simulink model "Backstep"  (R2015a)
settings: Solver=ode45  StartTime=0.0  StopTime=10.0  RelTol=1e-3
values from neighbouring files (symbols this model uses):
  a1 = (Iy-Iz)/Ix    (= -0.371382636656)    [Donnees_quadri.m]
  a2 = Irotor/Ix    (= 9.6463022508e-05)    [Donnees_quadri.m]
  a3 = (Iz-Ix)/Iy    (= 0.466575716235)    [Donnees_quadri.m]
  a4 = Irotor/Iy    (= 8.18553888131e-05)    [Donnees_quadri.m]
  a5 = (Ix-Iy)/Iz    (= -0.115145228216)    [Donnees_quadri.m]
  b1 = L/Ix    (= 16.077170418)    [Donnees_quadri.m]
  b2 = L/Iy    (= 13.6425648022)    [Donnees_quadri.m]
  b3 = L/Iz    (= 10.3734439834)    [Donnees_quadri.m]
  c1 = 5.52    [Donnees_quadri.m]
  c2 = 3.4    [Donnees_quadri.m]
  c3 = 1    [Donnees_quadri.m]
  c4 = 1    [Donnees_quadri.m]
  c5 = 3.07    [Donnees_quadri.m]
  c6 = 4.71    [Donnees_quadri.m]
  c7 = 6.11    [Donnees_quadri.m]
  c8 = 7.96    [Donnees_quadri.m]
  g = 9.81    [Donnees_quadri.m]
  m = 0.65    [Donnees_quadri.m]
  phi_dot_d = 0    [Donnees_quadri.m]
  psi_d = 2    [Donnees_quadri.m]
  psi_dot_d = 0    [Donnees_quadri.m]
  theta_dot_d = 0    [Donnees_quadri.m]
  x_dot_dot_d = 0    [Donnees_quadri.m]
  y_dot_dot_d = 0    [Donnees_quadri.m]
  z_d = 5    [Donnees_quadri.m]
  z_dot_d = 0    [Donnees_quadri.m]
settings Model: Creator=Lenovo  LastModifiedBy=Lenovo

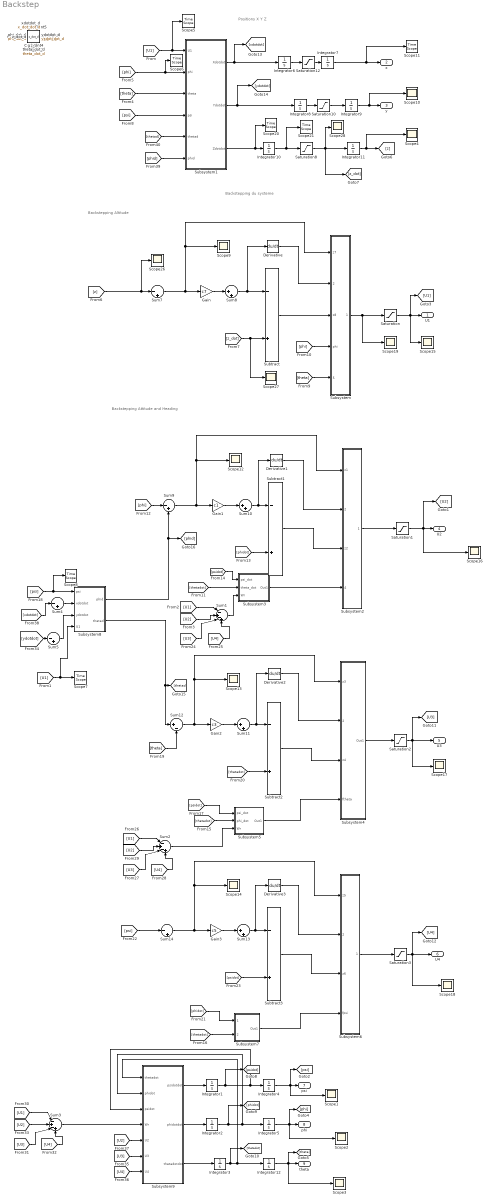
== system Backstep ==
  note: Positions X Y Z
  note: Backstepping Altitude
  note: Backstepping du systeme
  note: Backstepping Attitude and Heading
  Derivative{,1..3} (4 alike) : Derivative
  Gain : Gain  Gain=c7
  Gain1 : Gain  Gain=c1
  Gain2 : Gain  Gain=c3
  Gain3 : Gain  Gain=c5
  Integrator{1..12} (12 alike) : Integrator
  Saturation : Saturate  UpperLimit=500  LowerLimit=-500
  Saturation{1..3,8,10,12} (6 alike) : Saturate  UpperLimit=5  LowerLimit=-5
  Scope{1..4,9..10,12..19,26..28} (17 alike) : Scope
      Scope10 settings: SaveName=ScopeData9
      Scope12 settings: SaveName=ScopeData11
      Scope13 settings: SaveName=ScopeData12
      Scope14 settings: SaveName=ScopeData13
      Scope15 settings: SaveName=ScopeData14
      Scope16 settings: SaveName=ScopeData15
      Scope17 settings: SaveName=ScopeData16
      Scope18 settings: SaveName=ScopeData17
      Scope19 settings: SaveName=ScopeData24
      Scope2 settings: SaveName=ScopeData3
      Scope26 settings: SaveName=ScopeData39
      Scope27 settings: SaveName=ScopeData45
      Scope28 settings: SaveName=ScopeData46
      Scope3 settings: SaveName=ScopeData4
      Scope4 settings: SaveName=ScopeData2
      Scope9 settings: SaveName=ScopeData8
  Scope{5..8,11,20..21} (7 alike) : TimeScope
  Subsystem : Subsystem
  Subsystem1 : Subsystem
  Subsystem2 : Subsystem
  Subsystem3 : Subsystem
  Subsystem4 : Subsystem
  Subsystem5 : Subsystem
  Subsystem6 : Subsystem
  Subsystem7 : Subsystem
  Subsystem8 : Subsystem
  Subsystem9 : Subsystem
  Subtract{,1..3} (4 alike) : Sum  Inputs=-+
  Sum1 : Sum  Inputs=|-+-+
  Sum{8,10..11,13} (4 alike) : Sum  Inputs=|++
  Sum12 : Sum  Inputs=|+-
  Sum{4..5,7,9,14} (5 alike) : Sum  Inputs=|-+
  Sum2 : Sum  Inputs=|-+-+
  Sum3 : Sum  Inputs=|-+-+
  U1 : Outport
  x : Outport  Port=2
  y : Outport  Port=3
  U2 : Outport  Port=4
  U3 : Outport  Port=5
  U4 : Outport  Port=6
  psi : Outport  Port=7
  phi : Outport  Port=8
  "theta " : Outport  Port=9
  1 : Constant  IOType=siggen
  Constant : Constant  IOType=siggen
  Constant1 : Constant  IOType=siggen  Value=a4
  Constant2 : Constant  IOType=siggen  Value=a3
  Constant3 : Constant  IOType=siggen  Value=a2
  Constant4 : Constant  IOType=siggen  Value=a1
  Constant5 : Constant  IOType=siggen  Value=a5
  a1 : Constant  IOType=siggen  Value=a1
  a2 : Constant  IOType=siggen  Value=a2
  a3 : Constant  IOType=siggen  Value=a3
  a4 : Constant  IOType=siggen  Value=a4
  a5 : Constant  IOType=siggen  Value=a5
  b1 : Constant  IOType=siggen  Value=b1
  b2 : Constant  IOType=siggen  Value=b2
  b3 : Constant  IOType=siggen  Value=b3
  c2 : Constant  IOType=siggen  Value=c2
  c4 : Constant  IOType=siggen  Value=c4
  c6 : Constant  IOType=siggen  Value=c6
  c8 : Constant  IOType=siggen  Value=c8
  g : Constant  IOType=siggen  Value=g
  m : Constant  IOType=siggen  Value=m
  phi_dot_d : Constant  IOType=siggen  Value=phi_dot_d
  psi_d : Constant  IOType=siggen  Value=psi_d
  psi_dot_d : Constant  IOType=siggen  Value=psi_dot_d
  theta_dot_d : Constant  IOType=siggen  Value=theta_dot_d
  xdotdot_d : Constant  IOType=siggen  Value=x_dot_dot_d
  ydotdot_d : Constant  IOType=siggen  Value=y_dot_dot_d
  z_d : Constant  IOType=siggen  Value=z_d
  z_dot_d : Constant  IOType=siggen  Value=z_dot_d
  wires:
  Sum7/1 -> Scope9/1, Subsystem/1(z7), Gain/1
  Subtract/1 -> Subsystem/3(z8)
  Subsystem/1(Out1) -> Scope19/1, Saturation/1
  Gain/1 -> Sum8/1
  Sum8/1 -> Derivative/1, Subtract/1
  Saturation/1 -> [U1], Scope15/1, U1/1
  [U1] -> Scope5/1, Subsystem1/1(U1)
  Integrator6/1 -> Saturation12/1
  Integrator8/1 -> Saturation10/1
  Integrator10/1 -> Scope21/1, Saturation8/1
  Integrator11/1 -> Scope4/1, [z]
  [z] -> Scope26/1, Sum7/1
  Integrator9/1 -> Scope10/1, y/1
  Integrator7/1 -> Scope11/1, x/1
  Sum9/1 -> Scope12/1, Subsystem2/1(z1), Gain1/1
  Subtract1/1 -> Subsystem2/3(z2)
  Subsystem2/1(Out1) -> Saturation1/1
  Gain1/1 -> Sum10/1
  Sum10/1 -> Derivative1/1, Subtract1/1
  Saturation1/1 -> [U2], Scope16/1, U2/1
  Subsystem3/1(Out1) -> Subsystem2/4(fphi)
  [z_dot] -> Scope27/1, Subtract/2
  Sum12/1 -> Scope13/1, Subsystem4/1(z3), Gain2/1
  Subtract2/1 -> Subsystem4/3(z4)
  Subsystem4/1(Out1) -> Saturation2/1
  Gain2/1 -> Sum11/1
  Sum11/1 -> Derivative2/1, Subtract2/1
  Saturation2/1 -> [U3], Scope17/1, U3/1
  [psidot] -> Subsystem5/1(psi_dot)
  Subsystem5/1(Out1) -> Subsystem4/4(ftheta)
  [thetadot] -> Subtract2/2
  Sum14/1 -> Scope14/1, Subsystem6/1(z5), Gain3/1
  Subtract3/1 -> Subsystem6/3(z6)
  Subsystem6/1(Out1) -> Saturation3/1
  Gain3/1 -> Sum13/1
  Sum13/1 -> Derivative3/1, Subtract3/1
  Saturation3/1 -> [U4], U4/1, Scope18/1
  [phidot] -> Subsystem7/1(phi_dot)
  [thetadot] -> Subsystem7/2(theta_dot)
  Subsystem7/1(Out1) -> Subsystem6/4(fpsi)
  [psidot] -> Subtract3/2
  [phidot] -> Subtract1/2
  [theta] -> Subsystem/5(theta)
  Derivative/1 -> Subsystem/2(zdd_d+c7zd_d-c7zd)
  [phi] -> Subsystem/4(phi)
  Derivative1/1 -> Subsystem2/2(phidd_d+c1phid_d-c1phid)
  Derivative2/1 -> Subsystem4/2(thetadd_d+c3thetad_d-c3thetad)
  Derivative3/1 -> Subsystem6/2(psidd_d+c5psid_d-c5psid)
  Subsystem1/3(Zdotdot) -> Scope20/1, Integrator10/1
  Saturation8/1 -> Scope28/1, [z_dot], Integrator11/1
  Saturation10/1 -> Integrator9/1
  Subsystem1/2(Ydotdot) -> Integrator8/1, [ydotdot]
  Subsystem1/1(Xdotdot) -> Integrator6/1, [xdotdot]
  Saturation12/1 -> Integrator7/1
  [psi] -> Scope8/1, Subsystem8/1(psi)
  Subsystem8/1(phid) -> [phid], Sum9/2
  Subsystem8/2(thetad) -> [thetad], Sum12/1
  [U1] -> Subsystem8/4(U1), Scope7/1
  [thetadot] -> Subsystem5/2(phi_dot)
  [phi] -> Sum9/1
  [theta] -> Subsystem1/3(theta)
  [psi] -> Subsystem1/4(psi)
  [phi] -> Scope6/1, Subsystem1/2(phi)
  [U1] -> Sum1/1
  Sum1/1 -> Subsystem3/3(Wr)
  [U2] -> Sum1/2
  Subsystem9/2(phidotdot) -> Integrator2/1
  Subsystem9/1(psidotdot) -> Integrator1/1
  Subsystem9/3(thetadotdot) -> Integrator3/1
  Integrator4/1 -> Scope1/1, [psi], psi/1
  Integrator5/1 -> Scope2/1, [phi], phi/1
  Integrator12/1 -> Scope3/1, [theta], "theta "/1
  Integrator1/1 -> [psidot], Subsystem9/3(psidot), Integrator4/1
  Integrator2/1 -> [phidot], Subsystem9/2(phidot), Integrator5/1
  Integrator3/1 -> [thetadot], Subsystem9/1(thetadot), Integrator12/1
  [psidot] -> Subsystem3/1(psi_dot)
  [thetadot] -> Subsystem3/2(theta_dot)
  [theta] -> Sum12/2
  [psi] -> Sum14/1
  [U3] -> Sum1/3
  [U4] -> Sum1/4
  [U1] -> Sum2/1
  Sum2/1 -> Subsystem5/3(Wr)
  [U2] -> Sum2/2
  [U3] -> Sum2/3
  [U4] -> Sum2/4
  [U1] -> Sum3/1
  [U2] -> Sum3/2
  [U3] -> Sum3/3
  [U4] -> Sum3/4
  Sum3/1 -> Subsystem9/4(Wr)
  [U2] -> Subsystem9/5(U2)
  [U3] -> Subsystem9/6(U3)
  [U4] -> Subsystem9/7(U4)
  [thetad] -> Subsystem1/5(thetad)
  [phid] -> Subsystem1/6(phid)
  Sum4/1 -> Subsystem8/2(xdotdot)
  [ydotdot] -> Sum5/1
  Sum5/1 -> Subsystem8/3(ydotdot)
  [xdotdot] -> Sum4/1

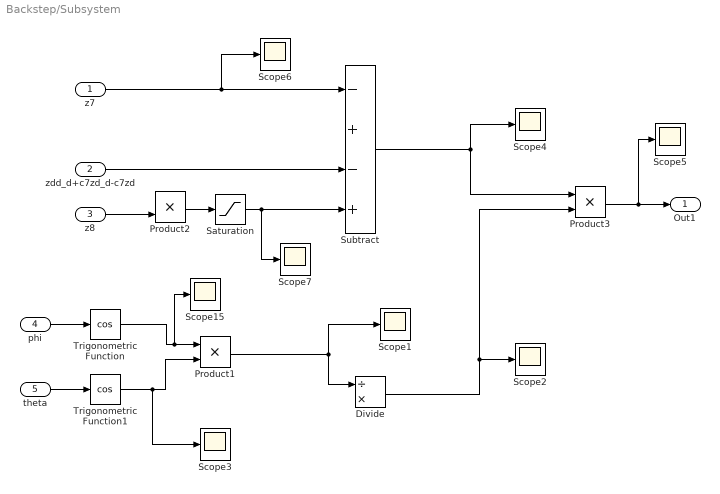
== system Backstep/Subsystem ==
  z7 : Inport
  zdd_d+c7zd_d-c7zd : Inport  Port=2
  z8 : Inport  Port=3
  phi : Inport  Port=4
  theta : Inport  Port=5
  Divide : Product  Inputs=/*
  Product1 : Product
  Product2 : Product
  Product3 : Product
  Saturation : Saturate  UpperLimit=5  LowerLimit=-5
  Scope{1..7,15} (8 alike) : Scope
      Scope1 settings: SaveName=ScopeData19
      Scope15 settings: SaveName=ScopeData18
      Scope2 settings: SaveName=ScopeData20
      Scope3 settings: SaveName=ScopeData21
      Scope4 settings: SaveName=ScopeData22
      Scope5 settings: SaveName=ScopeData23
      Scope6 settings: SaveName=ScopeData31
      Scope7 settings: SaveName=ScopeData32
  Subtract : Sum  Inputs=-+-+
  Trigonometric Function : Trigonometry  Operator=cos
  Trigonometric Function1 : Trigonometry  Operator=cos
  Out1 : Outport
  wires:
  z7/1 -> Scope6/1, Subtract/1
  phi/1 -> Trigonometric Function/1
  theta/1 -> Trigonometric Function1/1
  Product1/1 -> Scope1/1, Divide/1
  Trigonometric Function/1 -> Scope15/1, Product1/1
  Trigonometric Function1/1 -> Scope3/1, Product1/2
  z8/1 -> Product2/2
  Product3/1 -> Scope5/1, Out1/1
  Divide/1 -> Scope2/1, Product3/2
  Subtract/1 -> Product3/1, Scope4/1
  zdd_d+c7zd_d-c7zd/1 -> Subtract/3
  Product2/1 -> Saturation/1
  Saturation/1 -> Scope7/1, Subtract/4

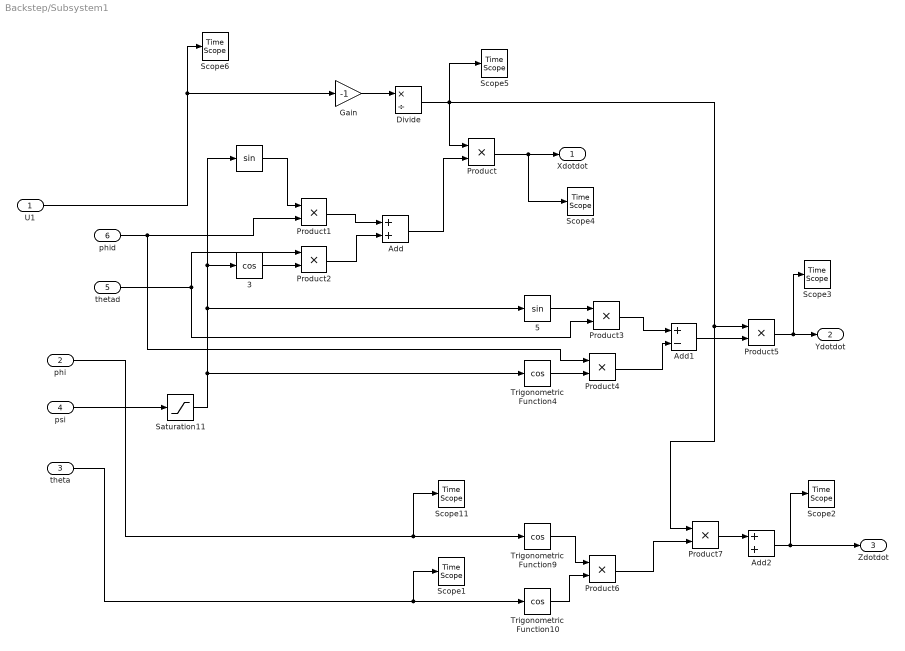
== system Backstep/Subsystem1 ==
  U1 : Inport
  phi : Inport  Port=2
  theta : Inport  Port=3
  psi : Inport  Port=4
  thetad : Inport  Port=5
  phid : Inport  Port=6
  " " : Trigonometry  ApproximationMethod=CORDIC
  3 : Trigonometry  Operator=cos  ApproximationMethod=CORDIC
  5 : Trigonometry  ApproximationMethod=CORDIC
  Add : Sum
  Add1 : Sum  Inputs=+-
  Add2 : Sum
  Divide : Product  Inputs=*/
  Gain : Gain  Gain=-1
  Product{,1..7} (8 alike) : Product
  Saturation11 : Saturate  UpperLimit=1  LowerLimit=-1
  Scope{1..6,11} (7 alike) : TimeScope
  Trigonometric Function10 : Trigonometry  Operator=cos  ApproximationMethod=CORDIC
  Trigonometric Function4 : Trigonometry  Operator=cos  ApproximationMethod=CORDIC
  Trigonometric Function9 : Trigonometry  Operator=cos  ApproximationMethod=CORDIC
  Xdotdot : Outport
  Ydotdot : Outport  Port=2
  Zdotdot : Outport  Port=3
  wires:
  Gain/1 -> Divide/1
  U1/1 -> Scope6/1, Gain/1
  Product/1 -> Scope4/1, Xdotdot/1
  Add/1 -> Product/2
  Product1/1 -> Add/1
  Product2/1 -> Add/2
  " "/1 -> Product1/1
  3/1 -> Product2/2
  phi/1 -> Scope11/1, Trigonometric Function9/1
  Product3/1 -> Add1/1
  Product4/1 -> Add1/2
  Product5/1 -> Scope3/1, Ydotdot/1
  Add1/1 -> Product5/2
  Divide/1 -> Scope5/1, Product/1, Product7/1, Product5/1
  theta/1 -> Scope1/1, Trigonometric Function10/1
  psi/1 -> Saturation11/1
  Add2/1 -> Scope2/1, Zdotdot/1
  Trigonometric Function10/1 -> Product6/2
  Trigonometric Function9/1 -> Product6/1
  Product7/1 -> Add2/1
  Product6/1 -> Product7/2
  5/1 -> Product3/1
  Trigonometric Function4/1 -> Product4/2
  Saturation11/1 -> 5/1, " "/1, 3/1, Trigonometric Function4/1
  thetad/1 -> Product3/2, Product2/1
  phid/1 -> Product4/1, Product1/2

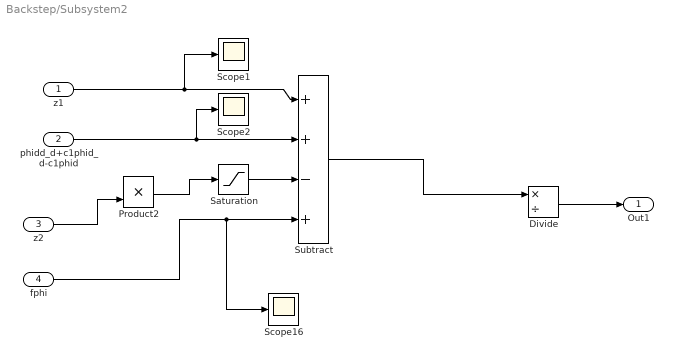
== system Backstep/Subsystem2 ==
  z1 : Inport
  phidd_d+c1phid_d-c1phid : Inport  Port=2
  z2 : Inport  Port=3
  fphi : Inport  Port=4
  Divide : Product  Inputs=*/
  Product2 : Product
  Saturation : Saturate  UpperLimit=5  LowerLimit=-5
  Scope1 : Scope
      settings: SaveName=ScopeData41
  Scope16 : Scope
      settings: SaveName=ScopeData40
  Scope2 : Scope
      settings: SaveName=ScopeData42
  Subtract : Sum  Inputs=++-+
  Out1 : Outport
  wires:
  z1/1 -> Scope1/1, Subtract/1
  z2/1 -> Product2/2
  Divide/1 -> Out1/1
  Subtract/1 -> Divide/1
  fphi/1 -> Scope16/1, Subtract/4
  Product2/1 -> Saturation/1
  phidd_d+c1phid_d-c1phid/1 -> Scope2/1, Subtract/2
  Saturation/1 -> Subtract/3

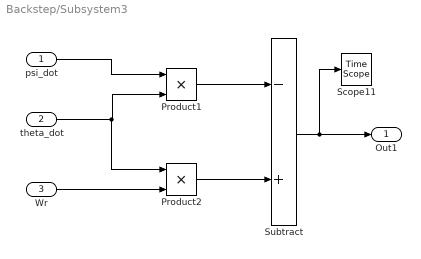
== system Backstep/Subsystem3 ==
  psi_dot : Inport
  theta_dot : Inport  Port=2
  Wr : Inport  Port=3
  Product1 : Product  Inputs=3
  Product2 : Product  Inputs=3
  Scope11 : TimeScope
  Subtract : Sum  Inputs=-+
  Out1 : Outport
  wires:
  psi_dot/1 -> Product1/1
  theta_dot/1 -> Product2/1, Product1/3
  Wr/1 -> Product2/3
  Product2/1 -> Subtract/2
  Product1/1 -> Subtract/1
  Subtract/1 -> Scope11/1, Out1/1

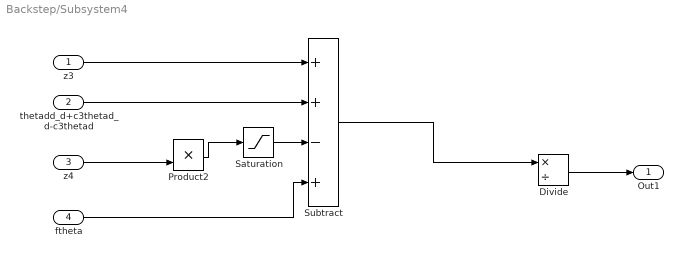
== system Backstep/Subsystem4 ==
  z3 : Inport
  thetadd_d+c3thetad_d-c3thetad : Inport  Port=2
  z4 : Inport  Port=3
  ftheta : Inport  Port=4
  Divide : Product  Inputs=*/
  Product2 : Product
  Saturation : Saturate  UpperLimit=5  LowerLimit=-5
  Subtract : Sum  Inputs=++-+
  Out1 : Outport
  wires:
  z3/1 -> Subtract/1
  ftheta/1 -> Subtract/4
  z4/1 -> Product2/2
  Divide/1 -> Out1/1
  Subtract/1 -> Divide/1
  thetadd_d+c3thetad_d-c3thetad/1 -> Subtract/2
  Product2/1 -> Saturation/1
  Saturation/1 -> Subtract/3

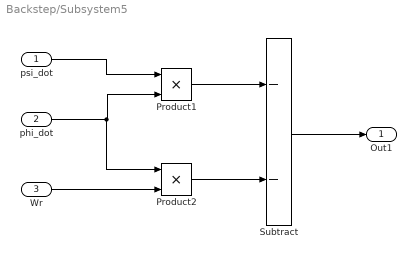
== system Backstep/Subsystem5 ==
  psi_dot : Inport
  phi_dot : Inport  Port=2
  Wr : Inport  Port=3
  Product1 : Product  Inputs=3
  Product2 : Product  Inputs=3
  Subtract : Sum  Inputs=--
  Out1 : Outport
  wires:
  psi_dot/1 -> Product1/1
  phi_dot/1 -> Product2/1, Product1/3
  Wr/1 -> Product2/3
  Product2/1 -> Subtract/2
  Product1/1 -> Subtract/1
  Subtract/1 -> Out1/1

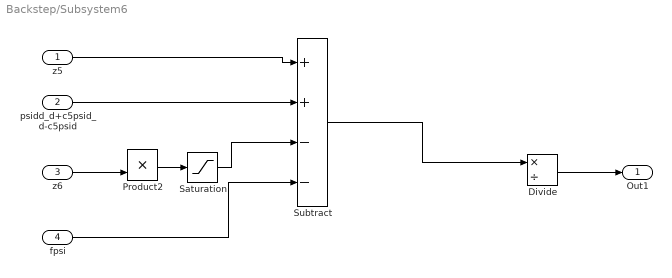
== system Backstep/Subsystem6 ==
  z5 : Inport
  psidd_d+c5psid_d-c5psid : Inport  Port=2
  z6 : Inport  Port=3
  fpsi : Inport  Port=4
  Divide : Product  Inputs=*/
  Product2 : Product
  Saturation : Saturate  UpperLimit=5  LowerLimit=-5
  Subtract : Sum  Inputs=++--
  Out1 : Outport
  wires:
  z5/1 -> Subtract/1
  z6/1 -> Product2/2
  Divide/1 -> Out1/1
  Subtract/1 -> Divide/1
  psidd_d+c5psid_d-c5psid/1 -> Subtract/2
  Product2/1 -> Saturation/1
  fpsi/1 -> Subtract/4
  Saturation/1 -> Subtract/3

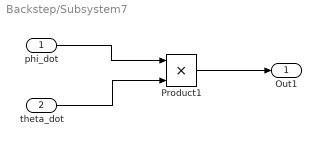
== system Backstep/Subsystem7 ==
  phi_dot : Inport
  theta_dot : Inport  Port=2
  Product1 : Product  Inputs=3
  Out1 : Outport
  wires:
  phi_dot/1 -> Product1/1
  theta_dot/1 -> Product1/3
  Product1/1 -> Out1/1

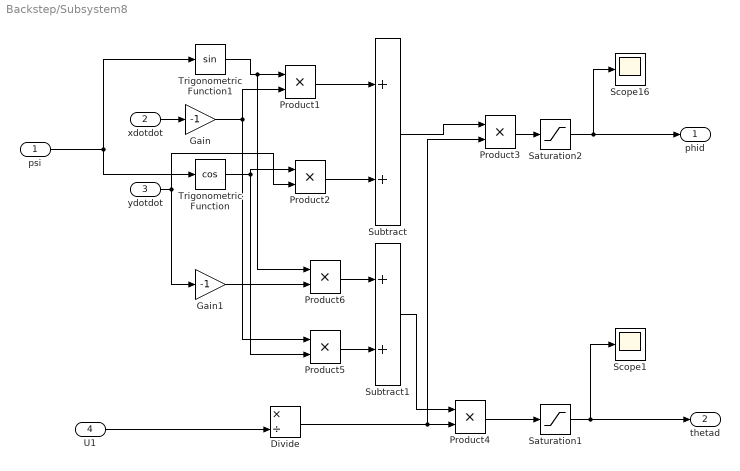
== system Backstep/Subsystem8 ==
  psi : Inport
  xdotdot : Inport  Port=2
  ydotdot : Inport  Port=3
  U1 : Inport  Port=4
  Divide : Product  Inputs=*/
  Gain : Gain  Gain=-1
  Gain1 : Gain  Gain=-1
  Product{1..6} (6 alike) : Product
  Saturation1 : Saturate  UpperLimit=20  LowerLimit=-20
  Saturation2 : Saturate  UpperLimit=20  LowerLimit=-20
  Scope1 : Scope
      settings: SaveName=ScopeData44
  Scope16 : Scope
      settings: SaveName=ScopeData43
  Subtract : Sum
  Subtract1 : Sum
  Trigonometric Function : Trigonometry  Operator=cos
  Trigonometric Function1 : Trigonometry
  phid : Outport
  thetad : Outport  Port=2
  wires:
  psi/1 -> Trigonometric Function1/1, Trigonometric Function/1
  Product2/1 -> Subtract/2
  Product1/1 -> Subtract/1
  xdotdot/1 -> Gain/1
  Gain/1 -> Product5/1, Product1/2
  Trigonometric Function1/1 -> Product6/1, Product1/1
  ydotdot/1 -> Gain1/1, Product2/2
  Trigonometric Function/1 -> Product5/2, Product2/1
  U1/1 -> Divide/2
  Product3/1 -> Saturation2/1
  Subtract/1 -> Product3/1
  Divide/1 -> Product4/2, Product3/2
  Product4/1 -> Saturation1/1
  Gain1/1 -> Product6/2
  Product5/1 -> Subtract1/2
  Product6/1 -> Subtract1/1
  Subtract1/1 -> Product4/1
  Saturation2/1 -> Scope16/1, phid/1
  Saturation1/1 -> Scope1/1, thetad/1

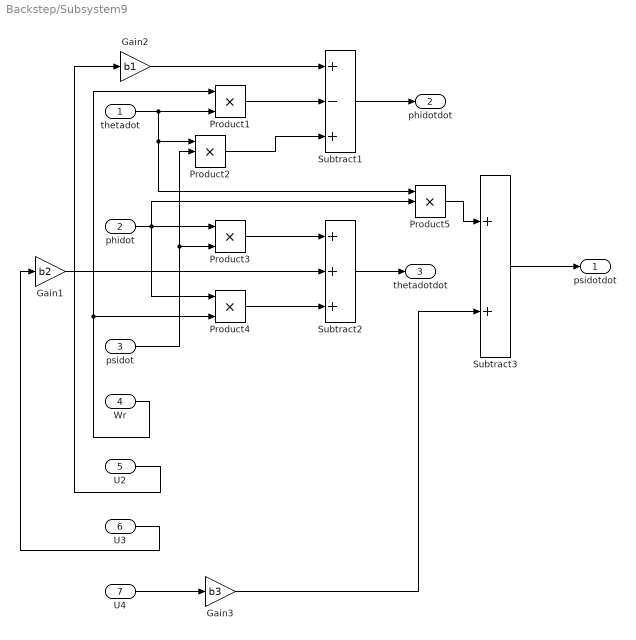
== system Backstep/Subsystem9 ==
  thetadot : Inport
  phidot : Inport  Port=2
  psidot : Inport  Port=3
  Wr : Inport  Port=4
  U2 : Inport  Port=5
  U3 : Inport  Port=6
  U4 : Inport  Port=7
  Gain1 : Gain  Gain=b2
  Gain2 : Gain  Gain=b1
  Gain3 : Gain  Gain=b3
  Product{1..5} (5 alike) : Product  Inputs=3
  Subtract1 : Sum  Inputs=+-+
  Subtract2 : Sum  Inputs=+++
  Subtract3 : Sum
  psidotdot : Outport
  phidotdot : Outport  Port=2
  thetadotdot : Outport  Port=3
  wires:
  thetadot/1 -> Product1/3, Product2/1, Product5/1
  psidot/1 -> Product3/3, Product2/2
  Wr/1 -> Product4/3, Product1/1
  U2/1 -> Gain2/1
  Product1/1 -> Subtract1/2
  Gain2/1 -> Subtract1/1
  Product2/1 -> Subtract1/3
  phidot/1 -> Product5/2, Product4/1, Product3/1
  Gain1/1 -> Subtract2/2
  Product3/1 -> Subtract2/1
  Product4/1 -> Subtract2/3
  U3/1 -> Gain1/1
  Product5/1 -> Subtract3/1
  U4/1 -> Gain3/1
  Gain3/1 -> Subtract3/2
  Subtract3/1 -> psidotdot/1
  Subtract1/1 -> phidotdot/1
  Subtract2/1 -> thetadotdot/1
